simulink model "Copy_of_tests"  (R2024b)
settings: Solver=VariableStepAuto  StartTime=0.0  StopTime=1  RelTol=1e-3  AbsTol=1e-3  EnableMultiTasking=on
values from neighbouring files (symbols this model uses):
  m = obj.Br *obj.volume / obj.mu    [External_Magnet2.m]
  Params = Sim_Param_Setup    [Sim_Open.m]
undefined symbols (not defined in the file or in its folder): X, Y, Z
libraries: sm_lib x171, vrlib x144, nesl_utility x101, matrix_library x91, sharedtransform x12
(part 5 of 9)

== system Copy_of_tests/Multi-Arm system/Single_Arm 1/Plate_2/Torques and Forces ==
  m_slave : Inport
  Pos_Slave : Inport  Port=2
  M1 : Inport  Port=3
  Pos_Plate1 : Inport  Port=4
  M3 : Inport  Port=5
  Pos_Plate3 : Inport  Port=6
  M4 : Inport  Port=7
  Pos_Plate4 : Inport  Port=8
  M5 : Inport  Port=9
  Pos_Plate5 : Inport  Port=10
  M6 : Inport  Port=11
  Pos_Plate6 : Inport  Port=12
  Add{,1..4} (5 alike) : Sum  Inputs=+-
  Magnetic Forces : Subsystem
  Magnetic Torques : Subsystem
      settings: PortSchema="{\"entries\":[{\"content\":{\"sides\":[{\"content\":{\"connectorIds\":[\"In1\",\"In2\",\"In3\",\"In4\",\"In5\",\"In6\",\"In7\",\"In8\",\"In9\",\"In10\",\"In11\"]},\"type\":\"ConnectorPlacement.EquallySpacedRectSide\",\"uuid\":\"6f05c61b-28f4-4565-bbea-1be0fb93c6f0\"},{\"content\":{\"connectorIds\":[\"Out1\"],\"side\":\"RIGHT\"},\"type\":\"ConnectorPlacement.EquallySpacedRectSide\",\"uuid\":\"8634642c-fc93-4182-aaec-4f6aca47cd70\"},{\"content\":{\"connectorIds\":[\"LConn1\"],\"side\":\"TOP\"},\"type\":\"ConnectorPlacement.EquallySpacedRectSide\",\"uuid\":\"4c29c46f-a8de-4915-ac6e-9828579e7b84\"}]},\"type\":\"ConnectorPlacement.EquallySpacedConnector\",\"uuid\":\"3da81916-5d74-4352-a0fa-851a5433a86b\"}],\"packageUris\":[\"http://schema.mathworks.com/mf0/Connector/R2020b\"],\"version\":\"1.0\"}"
  brick reference : PMIOPort  Side=Left
  Forces : Outport
  Torques : Outport  Port=2
  wires:
  m_slave/1 -> Magnetic Forces/1(m_slave), Magnetic Torques/1(m_slave)
  Pos_Slave/1 -> Add4/1, Add3/1, Add2/1, Add1/1, Add/1
  Pos_Plate1/1 -> Add/2
  M1/1 -> Magnetic Torques/2(M1), Magnetic Forces/2(M1)
  Add/1 -> Magnetic Torques/7(r1), Magnetic Forces/7(r1)
  Pos_Plate6/1 -> Add4/2
  Pos_Plate5/1 -> Add3/2
  Pos_Plate4/1 -> Add2/2
  Pos_Plate3/1 -> Add1/2
  M3/1 -> Magnetic Forces/3(M3), Magnetic Torques/3(M3)
  Add1/1 -> Magnetic Torques/8(r3), Magnetic Forces/8(r3)
  M4/1 -> Magnetic Forces/4(M4), Magnetic Torques/4(M4)
  M5/1 -> Magnetic Forces/5(M5), Magnetic Torques/5(M5)
  M6/1 -> Magnetic Forces/6(M6), Magnetic Torques/6(M6)
  Add2/1 -> Magnetic Forces/9(r4), Magnetic Torques/9(r4)
  Add3/1 -> Magnetic Forces/10(r5), Magnetic Torques/10(r5)
  Add4/1 -> Magnetic Forces/11(r6), Magnetic Torques/11(r6)
  Magnetic Forces/1(Forces) -> Forces/1
  Magnetic Torques/1(Torque) -> Torques/1
  connections:
  brick reference/RConn1 -- Magnetic Torques/LConn1

== system Copy_of_tests/Multi-Arm system/Single_Arm 1/Plate_3/Subsystem ==
  Slave_Moment : Inport
  Slave_Pos : Inport  Port=2
  Source_Moment : Inport  Port=3
  Source_Pos : Inport  Port=4
  Add : Sum  Inputs=+-
  Add1 : Sum  Inputs=+-
  Add2 : Sum  Inputs=+-
  Add3 : Sum  Inputs=+++
  Constant : Constant  Value=-3
  Constant1 : Constant  Value=-4
  Cross Product : matrix_library/Cross Product
  Dot Product : DotProduct  OutDataTypeStr=Inherit: Inherit via internal rule
  Dot Product1 : DotProduct  OutDataTypeStr=Inherit: Inherit via internal rule
  Gain : Gain  Gain=4*pi*1e-7/(4*pi)
  Gain1 : Gain  Gain=3
  Gain2 : Gain  Gain=3*4*pi*1e-7/(4*pi)
  Gain3 : Gain  Gain=5
  IdentityMatrix : IdentityMatrix  OutputDimensions=3
  Matrix Multiply : Product  Multiplication=Matrix(*)
  Matrix Multiply1 : Product  Multiplication=Matrix(*)
  Normalize Vector : vrlib/Utilities/Normalize Vector  maxzero=0
  Normalize Vector1 : vrlib/Utilities/Normalize Vector  maxzero=0
  Power : Math  Operator=pow
  Power1 : Math  Operator=pow
  Product{,1..5} (6 alike) : Product
  Sqrt : Sqrt
  Sqrt1 : Sqrt
  Transpose : Math  Operator=transpose
  m dot m : DotProduct  OutDataTypeStr=Inherit: Inherit via internal rule
  r dot m_master : DotProduct  OutDataTypeStr=Inherit: Inherit via internal rule
  r dot m_slave : DotProduct  OutDataTypeStr=Inherit: Inherit via internal rule
  Source_Torque : Outport
  Source_Force : Outport  Port=2
  wires:
  Power/1 -> Gain/1
  Transpose/1 -> Matrix Multiply/2
  Gain1/1 -> Add/1
  Matrix Multiply/1 -> Gain1/1
  Sqrt/1 -> Power/1
  Gain/1 -> Product/2
  Dot Product/1 -> Sqrt/1
  Product/1 -> Cross Product/2
  Matrix Multiply1/1 -> Product/1
  Normalize Vector/1 -> Transpose/1, Matrix Multiply/1
  IdentityMatrix/1 -> Add/2
  Constant/1 -> Power/2
  Add/1 -> Matrix Multiply1/1
  Slave_Pos/1 -> Add1/1
  Source_Pos/1 -> Add1/2
  Cross Product/1 -> Source_Torque/1
  Slave_Moment/1 -> Cross Product/1, Product2/2, m dot m/1, r dot m_slave/2
  Normalize Vector1/1 -> r dot m_slave/1, r dot m_master/1, Product4/2
  Add3/1 -> Product5/2
  Gain2/1 -> Product5/1
  Product4/1 -> Add3/3
  Dot Product1/1 -> Sqrt1/1
  Gain3/1 -> Add2/2
  r dot m_master/1 -> Product3/2, Product2/1
  Source_Moment/1 -> Matrix Multiply1/2, m dot m/2, Product1/2, r dot m_master/2
  m dot m/1 -> Add2/1
  Power1/1 -> Gain2/1
  Sqrt1/1 -> Power1/1
  r dot m_slave/1 -> Product1/1, Product3/1
  Product2/1 -> Add3/2
  Constant1/1 -> Power1/2
  Add2/1 -> Product4/1
  Add1/1 -> Normalize Vector1/1, Dot Product1/2, Dot Product1/1, Dot Product/2, Dot Product/1, Normalize Vector/1
  Product3/1 -> Gain3/1
  Product1/1 -> Add3/1
  Product5/1 -> Source_Force/1

== system Copy_of_tests/Multi-Arm system/Single_Arm 1/Plate_3/Torques and Forces ==
  m_slave : Inport
  Pos_Slave : Inport  Port=2
  M1 : Inport  Port=3
  Pos_Plate1 : Inport  Port=4
  M2 : Inport  Port=5
  Pos_Plate2 : Inport  Port=6
  M4 : Inport  Port=7
  Pos_Plate4 : Inport  Port=8
  M5 : Inport  Port=9
  Pos_Plate5 : Inport  Port=10
  M6 : Inport  Port=11
  Pos_Plate6 : Inport  Port=12
  Add{,1..4} (5 alike) : Sum  Inputs=+-
  Magnetic Forces : Subsystem
  Magnetic Torques : Subsystem
      settings: PortSchema="{\"entries\":[{\"content\":{\"sides\":[{\"content\":{\"connectorIds\":[\"In1\",\"In2\",\"In3\",\"In4\",\"In5\",\"In6\",\"In7\",\"In8\",\"In9\",\"In10\",\"In11\"]},\"type\":\"ConnectorPlacement.EquallySpacedRectSide\",\"uuid\":\"05771496-45a2-4580-b6ab-cadf9064ee26\"},{\"content\":{\"connectorIds\":[\"Out1\"],\"side\":\"RIGHT\"},\"type\":\"ConnectorPlacement.EquallySpacedRectSide\",\"uuid\":\"b79900f2-9f02-4790-af3a-0fbba66daa11\"},{\"content\":{\"connectorIds\":[\"LConn1\"],\"side\":\"TOP\"},\"type\":\"ConnectorPlacement.EquallySpacedRectSide\",\"uuid\":\"95266051-22b3-46d7-add2-de0ce2a92008\"}]},\"type\":\"ConnectorPlacement.EquallySpacedConnector\",\"uuid\":\"2bf1b23d-6512-437d-b945-3c726b6a255c\"}],\"packageUris\":[\"http://schema.mathworks.com/mf0/Connector/R2020b\"],\"version\":\"1.0\"}"
  brick reference : PMIOPort  Side=Left
  Forces : Outport
  Torques : Outport  Port=2
  wires:
  m_slave/1 -> Magnetic Forces/1(m_slave), Magnetic Torques/1(m_slave)
  Pos_Slave/1 -> Add4/1, Add3/1, Add2/1, Add1/1, Add/1
  Pos_Plate1/1 -> Add/2
  M1/1 -> Magnetic Torques/2(M1), Magnetic Forces/2(M1)
  Add/1 -> Magnetic Torques/7(r1), Magnetic Forces/7(r1)
  Pos_Plate6/1 -> Add4/2
  Pos_Plate5/1 -> Add3/2
  Pos_Plate4/1 -> Add2/2
  Pos_Plate2/1 -> Add1/2
  M2/1 -> Magnetic Forces/3(M2), Magnetic Torques/3(M2)
  Add1/1 -> Magnetic Torques/8(r2), Magnetic Forces/8(r2)
  M4/1 -> Magnetic Forces/4(M4), Magnetic Torques/4(M4)
  M5/1 -> Magnetic Forces/5(M5), Magnetic Torques/5(M5)
  M6/1 -> Magnetic Forces/6(M6), Magnetic Torques/6(M6)
  Add2/1 -> Magnetic Forces/9(r4), Magnetic Torques/9(r4)
  Add3/1 -> Magnetic Forces/10(r5), Magnetic Torques/10(r5)
  Add4/1 -> Magnetic Forces/11(r6), Magnetic Torques/11(r6)
  Magnetic Forces/1(Forces) -> Forces/1
  Magnetic Torques/1(Torque) -> Torques/1
  connections:
  brick reference/RConn1 -- Magnetic Torques/LConn1

== system Copy_of_tests/Multi-Arm system/Single_Arm 1/Plate_4/Subsystem ==
  Slave_Moment : Inport
  Slave_Pos : Inport  Port=2
  Source_Moment : Inport  Port=3
  Source_Pos : Inport  Port=4
  Add : Sum  Inputs=+-
  Add1 : Sum  Inputs=+-
  Add2 : Sum  Inputs=+-
  Add3 : Sum  Inputs=+++
  Constant : Constant  Value=-3
  Constant1 : Constant  Value=-4
  Cross Product : matrix_library/Cross Product
  Dot Product : DotProduct  OutDataTypeStr=Inherit: Inherit via internal rule
  Dot Product1 : DotProduct  OutDataTypeStr=Inherit: Inherit via internal rule
  Gain : Gain  Gain=4*pi*1e-7/(4*pi)
  Gain1 : Gain  Gain=3
  Gain2 : Gain  Gain=3*4*pi*1e-7/(4*pi)
  Gain3 : Gain  Gain=5
  IdentityMatrix : IdentityMatrix  OutputDimensions=3
  Matrix Multiply : Product  Multiplication=Matrix(*)
  Matrix Multiply1 : Product  Multiplication=Matrix(*)
  Normalize Vector : vrlib/Utilities/Normalize Vector  maxzero=0
  Normalize Vector1 : vrlib/Utilities/Normalize Vector  maxzero=0
  Power : Math  Operator=pow
  Power1 : Math  Operator=pow
  Product{,1..5} (6 alike) : Product
  Sqrt : Sqrt
  Sqrt1 : Sqrt
  Transpose : Math  Operator=transpose
  m dot m : DotProduct  OutDataTypeStr=Inherit: Inherit via internal rule
  r dot m_master : DotProduct  OutDataTypeStr=Inherit: Inherit via internal rule
  r dot m_slave : DotProduct  OutDataTypeStr=Inherit: Inherit via internal rule
  Source_Torque : Outport
  Source_Force : Outport  Port=2
  wires:
  Power/1 -> Gain/1
  Transpose/1 -> Matrix Multiply/2
  Gain1/1 -> Add/1
  Matrix Multiply/1 -> Gain1/1
  Sqrt/1 -> Power/1
  Gain/1 -> Product/2
  Dot Product/1 -> Sqrt/1
  Product/1 -> Cross Product/2
  Matrix Multiply1/1 -> Product/1
  Normalize Vector/1 -> Transpose/1, Matrix Multiply/1
  IdentityMatrix/1 -> Add/2
  Constant/1 -> Power/2
  Add/1 -> Matrix Multiply1/1
  Slave_Pos/1 -> Add1/1
  Source_Pos/1 -> Add1/2
  Cross Product/1 -> Source_Torque/1
  Slave_Moment/1 -> Cross Product/1, Product2/2, m dot m/1, r dot m_slave/2
  Normalize Vector1/1 -> r dot m_slave/1, r dot m_master/1, Product4/2
  Add3/1 -> Product5/2
  Gain2/1 -> Product5/1
  Product4/1 -> Add3/3
  Dot Product1/1 -> Sqrt1/1
  Gain3/1 -> Add2/2
  r dot m_master/1 -> Product3/2, Product2/1
  Source_Moment/1 -> Matrix Multiply1/2, m dot m/2, Product1/2, r dot m_master/2
  m dot m/1 -> Add2/1
  Power1/1 -> Gain2/1
  Sqrt1/1 -> Power1/1
  r dot m_slave/1 -> Product1/1, Product3/1
  Product2/1 -> Add3/2
  Constant1/1 -> Power1/2
  Add2/1 -> Product4/1
  Add1/1 -> Normalize Vector1/1, Dot Product1/2, Dot Product1/1, Dot Product/2, Dot Product/1, Normalize Vector/1
  Product3/1 -> Gain3/1
  Product1/1 -> Add3/1
  Product5/1 -> Source_Force/1

== system Copy_of_tests/Multi-Arm system/Single_Arm 1/Plate_4/Torques and Forces ==
  m_slave : Inport
  Pos_Slave : Inport  Port=2
  M1 : Inport  Port=3
  Pos_Plate1 : Inport  Port=4
  M2 : Inport  Port=5
  Pos_Plate2 : Inport  Port=6
  M3 : Inport  Port=7
  Pos_Plate3 : Inport  Port=8
  M5 : Inport  Port=9
  Pos_Plate5 : Inport  Port=10
  M6 : Inport  Port=11
  Pos_Plate6 : Inport  Port=12
  Add{,1..4} (5 alike) : Sum  Inputs=+-
  Magnetic Forces : Subsystem
  Magnetic Torques : Subsystem
      settings: PortSchema="{\"entries\":[{\"content\":{\"sides\":[{\"content\":{\"connectorIds\":[\"In1\",\"In2\",\"In3\",\"In4\",\"In5\",\"In6\",\"In7\",\"In8\",\"In9\",\"In10\",\"In11\"]},\"type\":\"ConnectorPlacement.EquallySpacedRectSide\",\"uuid\":\"05771496-45a2-4580-b6ab-cadf9064ee26\"},{\"content\":{\"connectorIds\":[\"Out1\"],\"side\":\"RIGHT\"},\"type\":\"ConnectorPlacement.EquallySpacedRectSide\",\"uuid\":\"b79900f2-9f02-4790-af3a-0fbba66daa11\"},{\"content\":{\"connectorIds\":[\"LConn1\"],\"side\":\"TOP\"},\"type\":\"ConnectorPlacement.EquallySpacedRectSide\",\"uuid\":\"95266051-22b3-46d7-add2-de0ce2a92008\"}]},\"type\":\"ConnectorPlacement.EquallySpacedConnector\",\"uuid\":\"2bf1b23d-6512-437d-b945-3c726b6a255c\"}],\"packageUris\":[\"http://schema.mathworks.com/mf0/Connector/R2020b\"],\"version\":\"1.0\"}"
  brick reference : PMIOPort  Side=Left
  Forces : Outport
  Torques : Outport  Port=2
  wires:
  m_slave/1 -> Magnetic Forces/1(m_slave), Magnetic Torques/1(m_slave)
  Pos_Slave/1 -> Add4/1, Add3/1, Add2/1, Add1/1, Add/1
  Pos_Plate1/1 -> Add/2
  M1/1 -> Magnetic Torques/2(M1), Magnetic Forces/2(M1)
  Add/1 -> Magnetic Torques/7(r1), Magnetic Forces/7(r1)
  Pos_Plate6/1 -> Add4/2
  Pos_Plate5/1 -> Add3/2
  Pos_Plate3/1 -> Add2/2
  Pos_Plate2/1 -> Add1/2
  M2/1 -> Magnetic Forces/3(M2), Magnetic Torques/3(M2)
  Add1/1 -> Magnetic Torques/8(r2), Magnetic Forces/8(r2)
  M3/1 -> Magnetic Forces/4(M3), Magnetic Torques/4(M3)
  M5/1 -> Magnetic Forces/5(M5), Magnetic Torques/5(M5)
  M6/1 -> Magnetic Forces/6(M6), Magnetic Torques/6(M6)
  Add2/1 -> Magnetic Forces/9(r3), Magnetic Torques/9(r3)
  Add3/1 -> Magnetic Forces/10(r5), Magnetic Torques/10(r5)
  Add4/1 -> Magnetic Forces/11(r6), Magnetic Torques/11(r6)
  Magnetic Forces/1(Forces) -> Forces/1
  Magnetic Torques/1(Torque) -> Torques/1
  connections:
  brick reference/RConn1 -- Magnetic Torques/LConn1

== system Copy_of_tests/Multi-Arm system/Single_Arm 1/Plate_5/Subsystem ==
  Slave_Moment : Inport
  Slave_Pos : Inport  Port=2
  Source_Moment : Inport  Port=3
  Source_Pos : Inport  Port=4
  Add : Sum  Inputs=+-
  Add1 : Sum  Inputs=+-
  Add2 : Sum  Inputs=+-
  Add3 : Sum  Inputs=+++
  Constant : Constant  Value=-3
  Constant1 : Constant  Value=-4
  Cross Product : matrix_library/Cross Product
  Dot Product : DotProduct  OutDataTypeStr=Inherit: Inherit via internal rule
  Dot Product1 : DotProduct  OutDataTypeStr=Inherit: Inherit via internal rule
  Gain : Gain  Gain=4*pi*1e-7/(4*pi)
  Gain1 : Gain  Gain=3
  Gain2 : Gain  Gain=3*4*pi*1e-7/(4*pi)
  Gain3 : Gain  Gain=5
  IdentityMatrix : IdentityMatrix  OutputDimensions=3
  Matrix Multiply : Product  Multiplication=Matrix(*)
  Matrix Multiply1 : Product  Multiplication=Matrix(*)
  Normalize Vector : vrlib/Utilities/Normalize Vector  maxzero=0
  Normalize Vector1 : vrlib/Utilities/Normalize Vector  maxzero=0
  Power : Math  Operator=pow
  Power1 : Math  Operator=pow
  Product{,1..5} (6 alike) : Product
  Sqrt : Sqrt
  Sqrt1 : Sqrt
  Transpose : Math  Operator=transpose
  m dot m : DotProduct  OutDataTypeStr=Inherit: Inherit via internal rule
  r dot m_master : DotProduct  OutDataTypeStr=Inherit: Inherit via internal rule
  r dot m_slave : DotProduct  OutDataTypeStr=Inherit: Inherit via internal rule
  Source_Torque : Outport
  Source_Force : Outport  Port=2
  wires:
  Power/1 -> Gain/1
  Transpose/1 -> Matrix Multiply/2
  Gain1/1 -> Add/1
  Matrix Multiply/1 -> Gain1/1
  Sqrt/1 -> Power/1
  Gain/1 -> Product/2
  Dot Product/1 -> Sqrt/1
  Product/1 -> Cross Product/2
  Matrix Multiply1/1 -> Product/1
  Normalize Vector/1 -> Transpose/1, Matrix Multiply/1
  IdentityMatrix/1 -> Add/2
  Constant/1 -> Power/2
  Add/1 -> Matrix Multiply1/1
  Slave_Pos/1 -> Add1/1
  Source_Pos/1 -> Add1/2
  Cross Product/1 -> Source_Torque/1
  Slave_Moment/1 -> Cross Product/1, Product2/2, m dot m/1, r dot m_slave/2
  Normalize Vector1/1 -> r dot m_slave/1, r dot m_master/1, Product4/2
  Add3/1 -> Product5/2
  Gain2/1 -> Product5/1
  Product4/1 -> Add3/3
  Dot Product1/1 -> Sqrt1/1
  Gain3/1 -> Add2/2
  r dot m_master/1 -> Product3/2, Product2/1
  Source_Moment/1 -> Matrix Multiply1/2, m dot m/2, Product1/2, r dot m_master/2
  m dot m/1 -> Add2/1
  Power1/1 -> Gain2/1
  Sqrt1/1 -> Power1/1
  r dot m_slave/1 -> Product1/1, Product3/1
  Product2/1 -> Add3/2
  Constant1/1 -> Power1/2
  Add2/1 -> Product4/1
  Add1/1 -> Normalize Vector1/1, Dot Product1/2, Dot Product1/1, Dot Product/2, Dot Product/1, Normalize Vector/1
  Product3/1 -> Gain3/1
  Product1/1 -> Add3/1
  Product5/1 -> Source_Force/1

== system Copy_of_tests/Multi-Arm system/Single_Arm 1/Plate_5/Torques and Forces ==
  m_slave : Inport
  Pos_Slave : Inport  Port=2
  M1 : Inport  Port=3
  Pos_Plate1 : Inport  Port=4
  M2 : Inport  Port=5
  Pos_Plate2 : Inport  Port=6
  M3 : Inport  Port=7
  Pos_Plate3 : Inport  Port=8
  M4 : Inport  Port=9
  Pos_Plate4 : Inport  Port=10
  M6 : Inport  Port=11
  Pos_Plate6 : Inport  Port=12
  Add{,1..4} (5 alike) : Sum  Inputs=+-
  Magnetic Forces : Subsystem
  Magnetic Torques : Subsystem
      settings: PortSchema="{\"entries\":[{\"content\":{\"sides\":[{\"content\":{\"connectorIds\":[\"In1\",\"In2\",\"In3\",\"In4\",\"In5\",\"In6\",\"In7\",\"In8\",\"In9\",\"In10\",\"In11\"]},\"type\":\"ConnectorPlacement.EquallySpacedRectSide\",\"uuid\":\"05771496-45a2-4580-b6ab-cadf9064ee26\"},{\"content\":{\"connectorIds\":[\"Out1\"],\"side\":\"RIGHT\"},\"type\":\"ConnectorPlacement.EquallySpacedRectSide\",\"uuid\":\"b79900f2-9f02-4790-af3a-0fbba66daa11\"},{\"content\":{\"connectorIds\":[\"LConn1\"],\"side\":\"TOP\"},\"type\":\"ConnectorPlacement.EquallySpacedRectSide\",\"uuid\":\"95266051-22b3-46d7-add2-de0ce2a92008\"}]},\"type\":\"ConnectorPlacement.EquallySpacedConnector\",\"uuid\":\"2bf1b23d-6512-437d-b945-3c726b6a255c\"}],\"packageUris\":[\"http://schema.mathworks.com/mf0/Connector/R2020b\"],\"version\":\"1.0\"}"
  brick reference : PMIOPort  Side=Left
  Forces : Outport
  Torques : Outport  Port=2
  wires:
  m_slave/1 -> Magnetic Forces/1(m_slave), Magnetic Torques/1(m_slave)
  Pos_Slave/1 -> Add4/1, Add3/1, Add2/1, Add1/1, Add/1
  Pos_Plate1/1 -> Add/2
  M1/1 -> Magnetic Torques/2(M1), Magnetic Forces/2(M1)
  Add/1 -> Magnetic Torques/7(r1), Magnetic Forces/7(r1)
  Pos_Plate6/1 -> Add4/2
  Pos_Plate4/1 -> Add3/2
  Pos_Plate3/1 -> Add2/2
  Pos_Plate2/1 -> Add1/2
  M2/1 -> Magnetic Forces/3(M2), Magnetic Torques/3(M2)
  Add1/1 -> Magnetic Torques/8(r2), Magnetic Forces/8(r2)
  M3/1 -> Magnetic Forces/4(M3), Magnetic Torques/4(M3)
  M4/1 -> Magnetic Forces/5(M4), Magnetic Torques/5(M4)
  M6/1 -> Magnetic Forces/6(M6), Magnetic Torques/6(M6)
  Add2/1 -> Magnetic Forces/9(r3), Magnetic Torques/9(r3)
  Add3/1 -> Magnetic Forces/10(r4), Magnetic Torques/10(r4)
  Add4/1 -> Magnetic Forces/11(r6), Magnetic Torques/11(r6)
  Magnetic Forces/1(Forces) -> Forces/1
  Magnetic Torques/1(Torque) -> Torques/1
  connections:
  brick reference/RConn1 -- Magnetic Torques/LConn1

== system Copy_of_tests/Multi-Arm system/Single_Arm 1/Plate_6/Subsystem ==
  Slave_Moment : Inport
  Slave_Pos : Inport  Port=2
  Source_Moment : Inport  Port=3
  Source_Pos : Inport  Port=4
  Add : Sum  Inputs=+-
  Add1 : Sum  Inputs=+-
  Add2 : Sum  Inputs=+-
  Add3 : Sum  Inputs=+++
  Constant : Constant  Value=-3
  Constant1 : Constant  Value=-4
  Cross Product : matrix_library/Cross Product
  Dot Product : DotProduct  OutDataTypeStr=Inherit: Inherit via internal rule
  Dot Product1 : DotProduct  OutDataTypeStr=Inherit: Inherit via internal rule
  Gain : Gain  Gain=4*pi*1e-7/(4*pi)
  Gain1 : Gain  Gain=3
  Gain2 : Gain  Gain=3*4*pi*1e-7/(4*pi)
  Gain3 : Gain  Gain=5
  IdentityMatrix : IdentityMatrix  OutputDimensions=3
  Matrix Multiply : Product  Multiplication=Matrix(*)
  Matrix Multiply1 : Product  Multiplication=Matrix(*)
  Normalize Vector : vrlib/Utilities/Normalize Vector  maxzero=0
  Normalize Vector1 : vrlib/Utilities/Normalize Vector  maxzero=0
  Power : Math  Operator=pow
  Power1 : Math  Operator=pow
  Product{,1..5} (6 alike) : Product
  Sqrt : Sqrt
  Sqrt1 : Sqrt
  Transpose : Math  Operator=transpose
  m dot m : DotProduct  OutDataTypeStr=Inherit: Inherit via internal rule
  r dot m_master : DotProduct  OutDataTypeStr=Inherit: Inherit via internal rule
  r dot m_slave : DotProduct  OutDataTypeStr=Inherit: Inherit via internal rule
  Source_Torque : Outport
  Source_Force : Outport  Port=2
  wires:
  Power/1 -> Gain/1
  Transpose/1 -> Matrix Multiply/2
  Gain1/1 -> Add/1
  Matrix Multiply/1 -> Gain1/1
  Sqrt/1 -> Power/1
  Gain/1 -> Product/2
  Dot Product/1 -> Sqrt/1
  Product/1 -> Cross Product/2
  Matrix Multiply1/1 -> Product/1
  Normalize Vector/1 -> Transpose/1, Matrix Multiply/1
  IdentityMatrix/1 -> Add/2
  Constant/1 -> Power/2
  Add/1 -> Matrix Multiply1/1
  Slave_Pos/1 -> Add1/1
  Source_Pos/1 -> Add1/2
  Cross Product/1 -> Source_Torque/1
  Slave_Moment/1 -> Cross Product/1, Product2/2, m dot m/1, r dot m_slave/2
  Normalize Vector1/1 -> r dot m_slave/1, r dot m_master/1, Product4/2
  Add3/1 -> Product5/2
  Gain2/1 -> Product5/1
  Product4/1 -> Add3/3
  Dot Product1/1 -> Sqrt1/1
  Gain3/1 -> Add2/2
  r dot m_master/1 -> Product3/2, Product2/1
  Source_Moment/1 -> Matrix Multiply1/2, m dot m/2, Product1/2, r dot m_master/2
  m dot m/1 -> Add2/1
  Power1/1 -> Gain2/1
  Sqrt1/1 -> Power1/1
  r dot m_slave/1 -> Product1/1, Product3/1
  Product2/1 -> Add3/2
  Constant1/1 -> Power1/2
  Add2/1 -> Product4/1
  Add1/1 -> Normalize Vector1/1, Dot Product1/2, Dot Product1/1, Dot Product/2, Dot Product/1, Normalize Vector/1
  Product3/1 -> Gain3/1
  Product1/1 -> Add3/1
  Product5/1 -> Source_Force/1

== system Copy_of_tests/Multi-Arm system/Single_Arm 1/Plate_6/Torques and Forces ==
  m_slave : Inport
  Pos_Slave : Inport  Port=2
  M1 : Inport  Port=3
  Pos_Plate1 : Inport  Port=4
  M2 : Inport  Port=5
  Pos_Plate2 : Inport  Port=6
  M3 : Inport  Port=7
  Pos_Plate3 : Inport  Port=8
  M4 : Inport  Port=9
  Pos_Plate4 : Inport  Port=10
  M5 : Inport  Port=11
  Pos_Plate5 : Inport  Port=12
  Add{,1..4} (5 alike) : Sum  Inputs=+-
  Magnetic Forces : Subsystem
  Magnetic Torques : Subsystem
      settings: PortSchema="{\"entries\":[{\"content\":{\"sides\":[{\"content\":{\"connectorIds\":[\"In1\",\"In2\",\"In3\",\"In4\",\"In5\",\"In6\",\"In7\",\"In8\",\"In9\",\"In10\",\"In11\"]},\"type\":\"ConnectorPlacement.EquallySpacedRectSide\",\"uuid\":\"6f05c61b-28f4-4565-bbea-1be0fb93c6f0\"},{\"content\":{\"connectorIds\":[\"Out1\"],\"side\":\"RIGHT\"},\"type\":\"ConnectorPlacement.EquallySpacedRectSide\",\"uuid\":\"8634642c-fc93-4182-aaec-4f6aca47cd70\"},{\"content\":{\"connectorIds\":[\"LConn1\"],\"side\":\"TOP\"},\"type\":\"ConnectorPlacement.EquallySpacedRectSide\",\"uuid\":\"4c29c46f-a8de-4915-ac6e-9828579e7b84\"}]},\"type\":\"ConnectorPlacement.EquallySpacedConnector\",\"uuid\":\"3da81916-5d74-4352-a0fa-851a5433a86b\"}],\"packageUris\":[\"http://schema.mathworks.com/mf0/Connector/R2020b\"],\"version\":\"1.0\"}"
  Brick reference : PMIOPort  Side=Left
  Forces : Outport
  Torques : Outport  Port=2
  wires:
  m_slave/1 -> Magnetic Forces/1(m_slave), Magnetic Torques/1(m_slave)
  Pos_Slave/1 -> Add4/1, Add3/1, Add2/1, Add1/1, Add/1
  Pos_Plate1/1 -> Add/2
  M1/1 -> Magnetic Torques/2(M1), Magnetic Forces/2(M1)
  Add/1 -> Magnetic Torques/7(r1), Magnetic Forces/7(r1)
  Pos_Plate5/1 -> Add4/2
  Pos_Plate4/1 -> Add3/2
  Pos_Plate3/1 -> Add2/2
  Pos_Plate2/1 -> Add1/2
  M2/1 -> Magnetic Forces/3(M2), Magnetic Torques/3(M2)
  Add1/1 -> Magnetic Torques/8(r2), Magnetic Forces/8(r2)
  M3/1 -> Magnetic Forces/4(M3), Magnetic Torques/4(M3)
  M4/1 -> Magnetic Forces/5(M4), Magnetic Torques/5(M4)
  M5/1 -> Magnetic Forces/6(M5), Magnetic Torques/6(M5)
  Add2/1 -> Magnetic Forces/9(r3), Magnetic Torques/9(r3)
  Add3/1 -> Magnetic Forces/10(r4), Magnetic Torques/10(r4)
  Add4/1 -> Magnetic Forces/11(r5), Magnetic Torques/11(r5)
  Magnetic Forces/1(Forces) -> Forces/1
  Magnetic Torques/1(Torque) -> Torques/1
  connections:
  Brick reference/RConn1 -- Magnetic Torques/LConn1

== system Copy_of_tests/Multi-Arm system/Single_Arm 2/Plate_1/Subsystem ==
  Slave_Moment : Inport
  Slave_Pos : Inport  Port=2
  Source_Moment : Inport  Port=3
  Source_Pos : Inport  Port=4
  Add : Sum  Inputs=+-
  Add1 : Sum  Inputs=+-
  Add2 : Sum  Inputs=+-
  Add3 : Sum  Inputs=+++
  Constant : Constant  Value=-3
  Constant1 : Constant  Value=-4
  Cross Product : matrix_library/Cross Product
  Dot Product : DotProduct  OutDataTypeStr=Inherit: Inherit via internal rule
  Dot Product1 : DotProduct  OutDataTypeStr=Inherit: Inherit via internal rule
  Gain : Gain  Gain=4*pi*1e-7/(4*pi)
  Gain1 : Gain  Gain=3
  Gain2 : Gain  Gain=3*4*pi*1e-7/(4*pi)
  Gain3 : Gain  Gain=5
  IdentityMatrix : IdentityMatrix  OutputDimensions=3
  Matrix Multiply : Product  Multiplication=Matrix(*)
  Matrix Multiply1 : Product  Multiplication=Matrix(*)
  Normalize Vector : vrlib/Utilities/Normalize Vector  maxzero=0
  Normalize Vector1 : vrlib/Utilities/Normalize Vector  maxzero=0
  Power : Math  Operator=pow
  Power1 : Math  Operator=pow
  Product{,1..5} (6 alike) : Product
  Sqrt : Sqrt
  Sqrt1 : Sqrt
  Transpose : Math  Operator=transpose
  m dot m : DotProduct  OutDataTypeStr=Inherit: Inherit via internal rule
  r dot m_master : DotProduct  OutDataTypeStr=Inherit: Inherit via internal rule
  r dot m_slave : DotProduct  OutDataTypeStr=Inherit: Inherit via internal rule
  Source_Torque : Outport
  Source_Force : Outport  Port=2
  wires:
  Power/1 -> Gain/1
  Transpose/1 -> Matrix Multiply/2
  Gain1/1 -> Add/1
  Matrix Multiply/1 -> Gain1/1
  Sqrt/1 -> Power/1
  Gain/1 -> Product/2
  Dot Product/1 -> Sqrt/1
  Product/1 -> Cross Product/2
  Matrix Multiply1/1 -> Product/1
  Normalize Vector/1 -> Transpose/1, Matrix Multiply/1
  IdentityMatrix/1 -> Add/2
  Constant/1 -> Power/2
  Add/1 -> Matrix Multiply1/1
  Slave_Pos/1 -> Add1/1
  Source_Pos/1 -> Add1/2
  Cross Product/1 -> Source_Torque/1
  Slave_Moment/1 -> Cross Product/1, Product2/2, m dot m/1, r dot m_slave/2
  Normalize Vector1/1 -> r dot m_slave/1, r dot m_master/1, Product4/2
  Add3/1 -> Product5/2
  Gain2/1 -> Product5/1
  Product4/1 -> Add3/3
  Dot Product1/1 -> Sqrt1/1
  Gain3/1 -> Add2/2
  r dot m_master/1 -> Product3/2, Product2/1
  Source_Moment/1 -> Matrix Multiply1/2, m dot m/2, Product1/2, r dot m_master/2
  m dot m/1 -> Add2/1
  Power1/1 -> Gain2/1
  Sqrt1/1 -> Power1/1
  r dot m_slave/1 -> Product1/1, Product3/1
  Product2/1 -> Add3/2
  Constant1/1 -> Power1/2
  Add2/1 -> Product4/1
  Add1/1 -> Normalize Vector1/1, Dot Product1/2, Dot Product1/1, Dot Product/2, Dot Product/1, Normalize Vector/1
  Product3/1 -> Gain3/1
  Product1/1 -> Add3/1
  Product5/1 -> Source_Force/1

== system Copy_of_tests/Multi-Arm system/Single_Arm 2/Plate_1/Torques and Forces ==
  m_slave : Inport
  Pos_Slave : Inport  Port=2
  M2 : Inport  Port=3
  Pos_Plate2 : Inport  Port=4
  M3 : Inport  Port=5
  Pos_Plate3 : Inport  Port=6
  M4 : Inport  Port=7
  Pos_Plate4 : Inport  Port=8
  M5 : Inport  Port=9
  Pos_Plate5 : Inport  Port=10
  M6 : Inport  Port=11
  Pos_Plate6 : Inport  Port=12
  Add{,1..4} (5 alike) : Sum  Inputs=+-
  Magnetic Forces : Subsystem
  Magnetic Torques : Subsystem
      settings: PortSchema="{\"entries\":[{\"content\":{\"sides\":[{\"content\":{\"connectorIds\":[\"In1\",\"In2\",\"In3\",\"In4\",\"In5\",\"In6\",\"In7\",\"In8\",\"In9\",\"In10\",\"In11\"]},\"type\":\"ConnectorPlacement.EquallySpacedRectSide\",\"uuid\":\"6f05c61b-28f4-4565-bbea-1be0fb93c6f0\"},{\"content\":{\"connectorIds\":[\"Out1\"],\"side\":\"RIGHT\"},\"type\":\"ConnectorPlacement.EquallySpacedRectSide\",\"uuid\":\"8634642c-fc93-4182-aaec-4f6aca47cd70\"},{\"content\":{\"connectorIds\":[\"LConn1\"],\"side\":\"TOP\"},\"type\":\"ConnectorPlacement.EquallySpacedRectSide\",\"uuid\":\"4c29c46f-a8de-4915-ac6e-9828579e7b84\"}]},\"type\":\"ConnectorPlacement.EquallySpacedConnector\",\"uuid\":\"3da81916-5d74-4352-a0fa-851a5433a86b\"}],\"packageUris\":[\"http://schema.mathworks.com/mf0/Connector/R2020b\"],\"version\":\"1.0\"}"
  brick reference : PMIOPort  Side=Left
  Forces : Outport
  Torques : Outport  Port=2
  wires:
  m_slave/1 -> Magnetic Forces/1(m_slave), Magnetic Torques/1(m_slave)
  Pos_Slave/1 -> Add4/1, Add3/1, Add2/1, Add1/1, Add/1
  Pos_Plate2/1 -> Add/2
  M2/1 -> Magnetic Torques/2(M2), Magnetic Forces/2(M2)
  Add/1 -> Magnetic Torques/7(r2), Magnetic Forces/7(r2)
  Pos_Plate6/1 -> Add4/2
  Pos_Plate5/1 -> Add3/2
  Pos_Plate4/1 -> Add2/2
  Pos_Plate3/1 -> Add1/2
  M3/1 -> Magnetic Forces/3(M3), Magnetic Torques/3(M3)
  Add1/1 -> Magnetic Torques/8(r3), Magnetic Forces/8(r3)
  M4/1 -> Magnetic Forces/4(M4), Magnetic Torques/4(M4)
  M5/1 -> Magnetic Forces/5(M5), Magnetic Torques/5(M5)
  M6/1 -> Magnetic Forces/6(M6), Magnetic Torques/6(M6)
  Add2/1 -> Magnetic Forces/9(r4), Magnetic Torques/9(r4)
  Add3/1 -> Magnetic Forces/10(r5), Magnetic Torques/10(r5)
  Add4/1 -> Magnetic Forces/11(r6), Magnetic Torques/11(r6)
  Magnetic Forces/1(Forces) -> Forces/1
  Magnetic Torques/1(Torque) -> Torques/1
  connections:
  brick reference/RConn1 -- Magnetic Torques/LConn1

== system Copy_of_tests/Multi-Arm system/Single_Arm 2/Plate_2/Subsystem ==
  Slave_Moment : Inport
  Slave_Pos : Inport  Port=2
  Source_Moment : Inport  Port=3
  Source_Pos : Inport  Port=4
  Add : Sum  Inputs=+-
  Add1 : Sum  Inputs=+-
  Add2 : Sum  Inputs=+-
  Add3 : Sum  Inputs=+++
  Constant : Constant  Value=-3
  Constant1 : Constant  Value=-4
  Cross Product : matrix_library/Cross Product
  Dot Product : DotProduct  OutDataTypeStr=Inherit: Inherit via internal rule
  Dot Product1 : DotProduct  OutDataTypeStr=Inherit: Inherit via internal rule
  Gain : Gain  Gain=4*pi*1e-7/(4*pi)
  Gain1 : Gain  Gain=3
  Gain2 : Gain  Gain=3*4*pi*1e-7/(4*pi)
  Gain3 : Gain  Gain=5
  IdentityMatrix : IdentityMatrix  OutputDimensions=3
  Matrix Multiply : Product  Multiplication=Matrix(*)
  Matrix Multiply1 : Product  Multiplication=Matrix(*)
  Normalize Vector : vrlib/Utilities/Normalize Vector  maxzero=0
  Normalize Vector1 : vrlib/Utilities/Normalize Vector  maxzero=0
  Power : Math  Operator=pow
  Power1 : Math  Operator=pow
  Product{,1..5} (6 alike) : Product
  Sqrt : Sqrt
  Sqrt1 : Sqrt
  Transpose : Math  Operator=transpose
  m dot m : DotProduct  OutDataTypeStr=Inherit: Inherit via internal rule
  r dot m_master : DotProduct  OutDataTypeStr=Inherit: Inherit via internal rule
  r dot m_slave : DotProduct  OutDataTypeStr=Inherit: Inherit via internal rule
  Source_Torque : Outport
  Source_Force : Outport  Port=2
  wires:
  Power/1 -> Gain/1
  Transpose/1 -> Matrix Multiply/2
  Gain1/1 -> Add/1
  Matrix Multiply/1 -> Gain1/1
  Sqrt/1 -> Power/1
  Gain/1 -> Product/2
  Dot Product/1 -> Sqrt/1
  Product/1 -> Cross Product/2
  Matrix Multiply1/1 -> Product/1
  Normalize Vector/1 -> Transpose/1, Matrix Multiply/1
  IdentityMatrix/1 -> Add/2
  Constant/1 -> Power/2
  Add/1 -> Matrix Multiply1/1
  Slave_Pos/1 -> Add1/1
  Source_Pos/1 -> Add1/2
  Cross Product/1 -> Source_Torque/1
  Slave_Moment/1 -> Cross Product/1, Product2/2, m dot m/1, r dot m_slave/2
  Normalize Vector1/1 -> r dot m_slave/1, r dot m_master/1, Product4/2
  Add3/1 -> Product5/2
  Gain2/1 -> Product5/1
  Product4/1 -> Add3/3
  Dot Product1/1 -> Sqrt1/1
  Gain3/1 -> Add2/2
  r dot m_master/1 -> Product3/2, Product2/1
  Source_Moment/1 -> Matrix Multiply1/2, m dot m/2, Product1/2, r dot m_master/2
  m dot m/1 -> Add2/1
  Power1/1 -> Gain2/1
  Sqrt1/1 -> Power1/1
  r dot m_slave/1 -> Product1/1, Product3/1
  Product2/1 -> Add3/2
  Constant1/1 -> Power1/2
  Add2/1 -> Product4/1
  Add1/1 -> Normalize Vector1/1, Dot Product1/2, Dot Product1/1, Dot Product/2, Dot Product/1, Normalize Vector/1
  Product3/1 -> Gain3/1
  Product1/1 -> Add3/1
  Product5/1 -> Source_Force/1

== system Copy_of_tests/Multi-Arm system/Single_Arm 2/Plate_2/Torques and Forces ==
  m_slave : Inport
  Pos_Slave : Inport  Port=2
  M1 : Inport  Port=3
  Pos_Plate1 : Inport  Port=4
  M3 : Inport  Port=5
  Pos_Plate3 : Inport  Port=6
  M4 : Inport  Port=7
  Pos_Plate4 : Inport  Port=8
  M5 : Inport  Port=9
  Pos_Plate5 : Inport  Port=10
  M6 : Inport  Port=11
  Pos_Plate6 : Inport  Port=12
  Add{,1..4} (5 alike) : Sum  Inputs=+-
  Magnetic Forces : Subsystem
  Magnetic Torques : Subsystem
      settings: PortSchema="{\"entries\":[{\"content\":{\"sides\":[{\"content\":{\"connectorIds\":[\"In1\",\"In2\",\"In3\",\"In4\",\"In5\",\"In6\",\"In7\",\"In8\",\"In9\",\"In10\",\"In11\"]},\"type\":\"ConnectorPlacement.EquallySpacedRectSide\",\"uuid\":\"6f05c61b-28f4-4565-bbea-1be0fb93c6f0\"},{\"content\":{\"connectorIds\":[\"Out1\"],\"side\":\"RIGHT\"},\"type\":\"ConnectorPlacement.EquallySpacedRectSide\",\"uuid\":\"8634642c-fc93-4182-aaec-4f6aca47cd70\"},{\"content\":{\"connectorIds\":[\"LConn1\"],\"side\":\"TOP\"},\"type\":\"ConnectorPlacement.EquallySpacedRectSide\",\"uuid\":\"4c29c46f-a8de-4915-ac6e-9828579e7b84\"}]},\"type\":\"ConnectorPlacement.EquallySpacedConnector\",\"uuid\":\"3da81916-5d74-4352-a0fa-851a5433a86b\"}],\"packageUris\":[\"http://schema.mathworks.com/mf0/Connector/R2020b\"],\"version\":\"1.0\"}"
  brick reference : PMIOPort  Side=Left
  Forces : Outport
  Torques : Outport  Port=2
  wires:
  m_slave/1 -> Magnetic Forces/1(m_slave), Magnetic Torques/1(m_slave)
  Pos_Slave/1 -> Add4/1, Add3/1, Add2/1, Add1/1, Add/1
  Pos_Plate1/1 -> Add/2
  M1/1 -> Magnetic Torques/2(M1), Magnetic Forces/2(M1)
  Add/1 -> Magnetic Torques/7(r1), Magnetic Forces/7(r1)
  Pos_Plate6/1 -> Add4/2
  Pos_Plate5/1 -> Add3/2
  Pos_Plate4/1 -> Add2/2
  Pos_Plate3/1 -> Add1/2
  M3/1 -> Magnetic Forces/3(M3), Magnetic Torques/3(M3)
  Add1/1 -> Magnetic Torques/8(r3), Magnetic Forces/8(r3)
  M4/1 -> Magnetic Forces/4(M4), Magnetic Torques/4(M4)
  M5/1 -> Magnetic Forces/5(M5), Magnetic Torques/5(M5)
  M6/1 -> Magnetic Forces/6(M6), Magnetic Torques/6(M6)
  Add2/1 -> Magnetic Forces/9(r4), Magnetic Torques/9(r4)
  Add3/1 -> Magnetic Forces/10(r5), Magnetic Torques/10(r5)
  Add4/1 -> Magnetic Forces/11(r6), Magnetic Torques/11(r6)
  Magnetic Forces/1(Forces) -> Forces/1
  Magnetic Torques/1(Torque) -> Torques/1
  connections:
  brick reference/RConn1 -- Magnetic Torques/LConn1

== system Copy_of_tests/Multi-Arm system/Single_Arm 2/Plate_3/Subsystem ==
  Slave_Moment : Inport
  Slave_Pos : Inport  Port=2
  Source_Moment : Inport  Port=3
  Source_Pos : Inport  Port=4
  Add : Sum  Inputs=+-
  Add1 : Sum  Inputs=+-
  Add2 : Sum  Inputs=+-
  Add3 : Sum  Inputs=+++
  Constant : Constant  Value=-3
  Constant1 : Constant  Value=-4
  Cross Product : matrix_library/Cross Product
  Dot Product : DotProduct  OutDataTypeStr=Inherit: Inherit via internal rule
  Dot Product1 : DotProduct  OutDataTypeStr=Inherit: Inherit via internal rule
  Gain : Gain  Gain=4*pi*1e-7/(4*pi)
  Gain1 : Gain  Gain=3
  Gain2 : Gain  Gain=3*4*pi*1e-7/(4*pi)
  Gain3 : Gain  Gain=5
  IdentityMatrix : IdentityMatrix  OutputDimensions=3
  Matrix Multiply : Product  Multiplication=Matrix(*)
  Matrix Multiply1 : Product  Multiplication=Matrix(*)
  Normalize Vector : vrlib/Utilities/Normalize Vector  maxzero=0
  Normalize Vector1 : vrlib/Utilities/Normalize Vector  maxzero=0
  Power : Math  Operator=pow
  Power1 : Math  Operator=pow
  Product{,1..5} (6 alike) : Product
  Sqrt : Sqrt
  Sqrt1 : Sqrt
  Transpose : Math  Operator=transpose
  m dot m : DotProduct  OutDataTypeStr=Inherit: Inherit via internal rule
  r dot m_master : DotProduct  OutDataTypeStr=Inherit: Inherit via internal rule
  r dot m_slave : DotProduct  OutDataTypeStr=Inherit: Inherit via internal rule
  Source_Torque : Outport
  Source_Force : Outport  Port=2
  wires:
  Power/1 -> Gain/1
  Transpose/1 -> Matrix Multiply/2
  Gain1/1 -> Add/1
  Matrix Multiply/1 -> Gain1/1
  Sqrt/1 -> Power/1
  Gain/1 -> Product/2
  Dot Product/1 -> Sqrt/1
  Product/1 -> Cross Product/2
  Matrix Multiply1/1 -> Product/1
  Normalize Vector/1 -> Transpose/1, Matrix Multiply/1
  IdentityMatrix/1 -> Add/2
  Constant/1 -> Power/2
  Add/1 -> Matrix Multiply1/1
  Slave_Pos/1 -> Add1/1
  Source_Pos/1 -> Add1/2
  Cross Product/1 -> Source_Torque/1
  Slave_Moment/1 -> Cross Product/1, Product2/2, m dot m/1, r dot m_slave/2
  Normalize Vector1/1 -> r dot m_slave/1, r dot m_master/1, Product4/2
  Add3/1 -> Product5/2
  Gain2/1 -> Product5/1
  Product4/1 -> Add3/3
  Dot Product1/1 -> Sqrt1/1
  Gain3/1 -> Add2/2
  r dot m_master/1 -> Product3/2, Product2/1
  Source_Moment/1 -> Matrix Multiply1/2, m dot m/2, Product1/2, r dot m_master/2
  m dot m/1 -> Add2/1
  Power1/1 -> Gain2/1
  Sqrt1/1 -> Power1/1
  r dot m_slave/1 -> Product1/1, Product3/1
  Product2/1 -> Add3/2
  Constant1/1 -> Power1/2
  Add2/1 -> Product4/1
  Add1/1 -> Normalize Vector1/1, Dot Product1/2, Dot Product1/1, Dot Product/2, Dot Product/1, Normalize Vector/1
  Product3/1 -> Gain3/1
  Product1/1 -> Add3/1
  Product5/1 -> Source_Force/1

== system Copy_of_tests/Multi-Arm system/Single_Arm 2/Plate_3/Torques and Forces ==
  m_slave : Inport
  Pos_Slave : Inport  Port=2
  M1 : Inport  Port=3
  Pos_Plate1 : Inport  Port=4
  M2 : Inport  Port=5
  Pos_Plate2 : Inport  Port=6
  M4 : Inport  Port=7
  Pos_Plate4 : Inport  Port=8
  M5 : Inport  Port=9
  Pos_Plate5 : Inport  Port=10
  M6 : Inport  Port=11
  Pos_Plate6 : Inport  Port=12
  Add{,1..4} (5 alike) : Sum  Inputs=+-
  Magnetic Forces : Subsystem
  Magnetic Torques : Subsystem
      settings: PortSchema="{\"entries\":[{\"content\":{\"sides\":[{\"content\":{\"connectorIds\":[\"In1\",\"In2\",\"In3\",\"In4\",\"In5\",\"In6\",\"In7\",\"In8\",\"In9\",\"In10\",\"In11\"]},\"type\":\"ConnectorPlacement.EquallySpacedRectSide\",\"uuid\":\"05771496-45a2-4580-b6ab-cadf9064ee26\"},{\"content\":{\"connectorIds\":[\"Out1\"],\"side\":\"RIGHT\"},\"type\":\"ConnectorPlacement.EquallySpacedRectSide\",\"uuid\":\"b79900f2-9f02-4790-af3a-0fbba66daa11\"},{\"content\":{\"connectorIds\":[\"LConn1\"],\"side\":\"TOP\"},\"type\":\"ConnectorPlacement.EquallySpacedRectSide\",\"uuid\":\"95266051-22b3-46d7-add2-de0ce2a92008\"}]},\"type\":\"ConnectorPlacement.EquallySpacedConnector\",\"uuid\":\"2bf1b23d-6512-437d-b945-3c726b6a255c\"}],\"packageUris\":[\"http://schema.mathworks.com/mf0/Connector/R2020b\"],\"version\":\"1.0\"}"
  brick reference : PMIOPort  Side=Left
  Forces : Outport
  Torques : Outport  Port=2
  wires:
  m_slave/1 -> Magnetic Forces/1(m_slave), Magnetic Torques/1(m_slave)
  Pos_Slave/1 -> Add4/1, Add3/1, Add2/1, Add1/1, Add/1
  Pos_Plate1/1 -> Add/2
  M1/1 -> Magnetic Torques/2(M1), Magnetic Forces/2(M1)
  Add/1 -> Magnetic Torques/7(r1), Magnetic Forces/7(r1)
  Pos_Plate6/1 -> Add4/2
  Pos_Plate5/1 -> Add3/2
  Pos_Plate4/1 -> Add2/2
  Pos_Plate2/1 -> Add1/2
  M2/1 -> Magnetic Forces/3(M2), Magnetic Torques/3(M2)
  Add1/1 -> Magnetic Torques/8(r2), Magnetic Forces/8(r2)
  M4/1 -> Magnetic Forces/4(M4), Magnetic Torques/4(M4)
  M5/1 -> Magnetic Forces/5(M5), Magnetic Torques/5(M5)
  M6/1 -> Magnetic Forces/6(M6), Magnetic Torques/6(M6)
  Add2/1 -> Magnetic Forces/9(r4), Magnetic Torques/9(r4)
  Add3/1 -> Magnetic Forces/10(r5), Magnetic Torques/10(r5)
  Add4/1 -> Magnetic Forces/11(r6), Magnetic Torques/11(r6)
  Magnetic Forces/1(Forces) -> Forces/1
  Magnetic Torques/1(Torque) -> Torques/1
  connections:
  brick reference/RConn1 -- Magnetic Torques/LConn1

== system Copy_of_tests/Multi-Arm system/Single_Arm 2/Plate_4/Subsystem ==
  Slave_Moment : Inport
  Slave_Pos : Inport  Port=2
  Source_Moment : Inport  Port=3
  Source_Pos : Inport  Port=4
  Add : Sum  Inputs=+-
  Add1 : Sum  Inputs=+-
  Add2 : Sum  Inputs=+-
  Add3 : Sum  Inputs=+++
  Constant : Constant  Value=-3
  Constant1 : Constant  Value=-4
  Cross Product : matrix_library/Cross Product
  Dot Product : DotProduct  OutDataTypeStr=Inherit: Inherit via internal rule
  Dot Product1 : DotProduct  OutDataTypeStr=Inherit: Inherit via internal rule
  Gain : Gain  Gain=4*pi*1e-7/(4*pi)
  Gain1 : Gain  Gain=3
  Gain2 : Gain  Gain=3*4*pi*1e-7/(4*pi)
  Gain3 : Gain  Gain=5
  IdentityMatrix : IdentityMatrix  OutputDimensions=3
  Matrix Multiply : Product  Multiplication=Matrix(*)
  Matrix Multiply1 : Product  Multiplication=Matrix(*)
  Normalize Vector : vrlib/Utilities/Normalize Vector  maxzero=0
  Normalize Vector1 : vrlib/Utilities/Normalize Vector  maxzero=0
  Power : Math  Operator=pow
  Power1 : Math  Operator=pow
  Product{,1..5} (6 alike) : Product
  Sqrt : Sqrt
  Sqrt1 : Sqrt
  Transpose : Math  Operator=transpose
  m dot m : DotProduct  OutDataTypeStr=Inherit: Inherit via internal rule
  r dot m_master : DotProduct  OutDataTypeStr=Inherit: Inherit via internal rule
  r dot m_slave : DotProduct  OutDataTypeStr=Inherit: Inherit via internal rule
  Source_Torque : Outport
  Source_Force : Outport  Port=2
  wires:
  Power/1 -> Gain/1
  Transpose/1 -> Matrix Multiply/2
  Gain1/1 -> Add/1
  Matrix Multiply/1 -> Gain1/1
  Sqrt/1 -> Power/1
  Gain/1 -> Product/2
  Dot Product/1 -> Sqrt/1
  Product/1 -> Cross Product/2
  Matrix Multiply1/1 -> Product/1
  Normalize Vector/1 -> Transpose/1, Matrix Multiply/1
  IdentityMatrix/1 -> Add/2
  Constant/1 -> Power/2
  Add/1 -> Matrix Multiply1/1
  Slave_Pos/1 -> Add1/1
  Source_Pos/1 -> Add1/2
  Cross Product/1 -> Source_Torque/1
  Slave_Moment/1 -> Cross Product/1, Product2/2, m dot m/1, r dot m_slave/2
  Normalize Vector1/1 -> r dot m_slave/1, r dot m_master/1, Product4/2
  Add3/1 -> Product5/2
  Gain2/1 -> Product5/1
  Product4/1 -> Add3/3
  Dot Product1/1 -> Sqrt1/1
  Gain3/1 -> Add2/2
  r dot m_master/1 -> Product3/2, Product2/1
  Source_Moment/1 -> Matrix Multiply1/2, m dot m/2, Product1/2, r dot m_master/2
  m dot m/1 -> Add2/1
  Power1/1 -> Gain2/1
  Sqrt1/1 -> Power1/1
  r dot m_slave/1 -> Product1/1, Product3/1
  Product2/1 -> Add3/2
  Constant1/1 -> Power1/2
  Add2/1 -> Product4/1
  Add1/1 -> Normalize Vector1/1, Dot Product1/2, Dot Product1/1, Dot Product/2, Dot Product/1, Normalize Vector/1
  Product3/1 -> Gain3/1
  Product1/1 -> Add3/1
  Product5/1 -> Source_Force/1

== system Copy_of_tests/Multi-Arm system/Single_Arm 2/Plate_4/Torques and Forces ==
  m_slave : Inport
  Pos_Slave : Inport  Port=2
  M1 : Inport  Port=3
  Pos_Plate1 : Inport  Port=4
  M2 : Inport  Port=5
  Pos_Plate2 : Inport  Port=6
  M3 : Inport  Port=7
  Pos_Plate3 : Inport  Port=8
  M5 : Inport  Port=9
  Pos_Plate5 : Inport  Port=10
  M6 : Inport  Port=11
  Pos_Plate6 : Inport  Port=12
  Add{,1..4} (5 alike) : Sum  Inputs=+-
  Magnetic Forces : Subsystem
  Magnetic Torques : Subsystem
      settings: PortSchema="{\"entries\":[{\"content\":{\"sides\":[{\"content\":{\"connectorIds\":[\"In1\",\"In2\",\"In3\",\"In4\",\"In5\",\"In6\",\"In7\",\"In8\",\"In9\",\"In10\",\"In11\"]},\"type\":\"ConnectorPlacement.EquallySpacedRectSide\",\"uuid\":\"05771496-45a2-4580-b6ab-cadf9064ee26\"},{\"content\":{\"connectorIds\":[\"Out1\"],\"side\":\"RIGHT\"},\"type\":\"ConnectorPlacement.EquallySpacedRectSide\",\"uuid\":\"b79900f2-9f02-4790-af3a-0fbba66daa11\"},{\"content\":{\"connectorIds\":[\"LConn1\"],\"side\":\"TOP\"},\"type\":\"ConnectorPlacement.EquallySpacedRectSide\",\"uuid\":\"95266051-22b3-46d7-add2-de0ce2a92008\"}]},\"type\":\"ConnectorPlacement.EquallySpacedConnector\",\"uuid\":\"2bf1b23d-6512-437d-b945-3c726b6a255c\"}],\"packageUris\":[\"http://schema.mathworks.com/mf0/Connector/R2020b\"],\"version\":\"1.0\"}"
  brick reference : PMIOPort  Side=Left
  Forces : Outport
  Torques : Outport  Port=2
  wires:
  m_slave/1 -> Magnetic Forces/1(m_slave), Magnetic Torques/1(m_slave)
  Pos_Slave/1 -> Add4/1, Add3/1, Add2/1, Add1/1, Add/1
  Pos_Plate1/1 -> Add/2
  M1/1 -> Magnetic Torques/2(M1), Magnetic Forces/2(M1)
  Add/1 -> Magnetic Torques/7(r1), Magnetic Forces/7(r1)
  Pos_Plate6/1 -> Add4/2
  Pos_Plate5/1 -> Add3/2
  Pos_Plate3/1 -> Add2/2
  Pos_Plate2/1 -> Add1/2
  M2/1 -> Magnetic Forces/3(M2), Magnetic Torques/3(M2)
  Add1/1 -> Magnetic Torques/8(r2), Magnetic Forces/8(r2)
  M3/1 -> Magnetic Forces/4(M3), Magnetic Torques/4(M3)
  M5/1 -> Magnetic Forces/5(M5), Magnetic Torques/5(M5)
  M6/1 -> Magnetic Forces/6(M6), Magnetic Torques/6(M6)
  Add2/1 -> Magnetic Forces/9(r3), Magnetic Torques/9(r3)
  Add3/1 -> Magnetic Forces/10(r5), Magnetic Torques/10(r5)
  Add4/1 -> Magnetic Forces/11(r6), Magnetic Torques/11(r6)
  Magnetic Forces/1(Forces) -> Forces/1
  Magnetic Torques/1(Torque) -> Torques/1
  connections:
  brick reference/RConn1 -- Magnetic Torques/LConn1

== system Copy_of_tests/Multi-Arm system/Single_Arm 2/Plate_5/Subsystem ==
  Slave_Moment : Inport
  Slave_Pos : Inport  Port=2
  Source_Moment : Inport  Port=3
  Source_Pos : Inport  Port=4
  Add : Sum  Inputs=+-
  Add1 : Sum  Inputs=+-
  Add2 : Sum  Inputs=+-
  Add3 : Sum  Inputs=+++
  Constant : Constant  Value=-3
  Constant1 : Constant  Value=-4
  Cross Product : matrix_library/Cross Product
  Dot Product : DotProduct  OutDataTypeStr=Inherit: Inherit via internal rule
  Dot Product1 : DotProduct  OutDataTypeStr=Inherit: Inherit via internal rule
  Gain : Gain  Gain=4*pi*1e-7/(4*pi)
  Gain1 : Gain  Gain=3
  Gain2 : Gain  Gain=3*4*pi*1e-7/(4*pi)
  Gain3 : Gain  Gain=5
  IdentityMatrix : IdentityMatrix  OutputDimensions=3
  Matrix Multiply : Product  Multiplication=Matrix(*)
  Matrix Multiply1 : Product  Multiplication=Matrix(*)
  Normalize Vector : vrlib/Utilities/Normalize Vector  maxzero=0
  Normalize Vector1 : vrlib/Utilities/Normalize Vector  maxzero=0
  Power : Math  Operator=pow
  Power1 : Math  Operator=pow
  Product{,1..5} (6 alike) : Product
  Sqrt : Sqrt
  Sqrt1 : Sqrt
  Transpose : Math  Operator=transpose
  m dot m : DotProduct  OutDataTypeStr=Inherit: Inherit via internal rule
  r dot m_master : DotProduct  OutDataTypeStr=Inherit: Inherit via internal rule
  r dot m_slave : DotProduct  OutDataTypeStr=Inherit: Inherit via internal rule
  Source_Torque : Outport
  Source_Force : Outport  Port=2
  wires:
  Power/1 -> Gain/1
  Transpose/1 -> Matrix Multiply/2
  Gain1/1 -> Add/1
  Matrix Multiply/1 -> Gain1/1
  Sqrt/1 -> Power/1
  Gain/1 -> Product/2
  Dot Product/1 -> Sqrt/1
  Product/1 -> Cross Product/2
  Matrix Multiply1/1 -> Product/1
  Normalize Vector/1 -> Transpose/1, Matrix Multiply/1
  IdentityMatrix/1 -> Add/2
  Constant/1 -> Power/2
  Add/1 -> Matrix Multiply1/1
  Slave_Pos/1 -> Add1/1
  Source_Pos/1 -> Add1/2
  Cross Product/1 -> Source_Torque/1
  Slave_Moment/1 -> Cross Product/1, Product2/2, m dot m/1, r dot m_slave/2
  Normalize Vector1/1 -> r dot m_slave/1, r dot m_master/1, Product4/2
  Add3/1 -> Product5/2
  Gain2/1 -> Product5/1
  Product4/1 -> Add3/3
  Dot Product1/1 -> Sqrt1/1
  Gain3/1 -> Add2/2
  r dot m_master/1 -> Product3/2, Product2/1
  Source_Moment/1 -> Matrix Multiply1/2, m dot m/2, Product1/2, r dot m_master/2
  m dot m/1 -> Add2/1
  Power1/1 -> Gain2/1
  Sqrt1/1 -> Power1/1
  r dot m_slave/1 -> Product1/1, Product3/1
  Product2/1 -> Add3/2
  Constant1/1 -> Power1/2
  Add2/1 -> Product4/1
  Add1/1 -> Normalize Vector1/1, Dot Product1/2, Dot Product1/1, Dot Product/2, Dot Product/1, Normalize Vector/1
  Product3/1 -> Gain3/1
  Product1/1 -> Add3/1
  Product5/1 -> Source_Force/1

== system Copy_of_tests/Multi-Arm system/Single_Arm 2/Plate_5/Torques and Forces ==
  m_slave : Inport
  Pos_Slave : Inport  Port=2
  M1 : Inport  Port=3
  Pos_Plate1 : Inport  Port=4
  M2 : Inport  Port=5
  Pos_Plate2 : Inport  Port=6
  M3 : Inport  Port=7
  Pos_Plate3 : Inport  Port=8
  M4 : Inport  Port=9
  Pos_Plate4 : Inport  Port=10
  M6 : Inport  Port=11
  Pos_Plate6 : Inport  Port=12
  Add{,1..4} (5 alike) : Sum  Inputs=+-
  Magnetic Forces : Subsystem
  Magnetic Torques : Subsystem
      settings: PortSchema="{\"entries\":[{\"content\":{\"sides\":[{\"content\":{\"connectorIds\":[\"In1\",\"In2\",\"In3\",\"In4\",\"In5\",\"In6\",\"In7\",\"In8\",\"In9\",\"In10\",\"In11\"]},\"type\":\"ConnectorPlacement.EquallySpacedRectSide\",\"uuid\":\"05771496-45a2-4580-b6ab-cadf9064ee26\"},{\"content\":{\"connectorIds\":[\"Out1\"],\"side\":\"RIGHT\"},\"type\":\"ConnectorPlacement.EquallySpacedRectSide\",\"uuid\":\"b79900f2-9f02-4790-af3a-0fbba66daa11\"},{\"content\":{\"connectorIds\":[\"LConn1\"],\"side\":\"TOP\"},\"type\":\"ConnectorPlacement.EquallySpacedRectSide\",\"uuid\":\"95266051-22b3-46d7-add2-de0ce2a92008\"}]},\"type\":\"ConnectorPlacement.EquallySpacedConnector\",\"uuid\":\"2bf1b23d-6512-437d-b945-3c726b6a255c\"}],\"packageUris\":[\"http://schema.mathworks.com/mf0/Connector/R2020b\"],\"version\":\"1.0\"}"
  brick reference : PMIOPort  Side=Left
  Forces : Outport
  Torques : Outport  Port=2
  wires:
  m_slave/1 -> Magnetic Forces/1(m_slave), Magnetic Torques/1(m_slave)
  Pos_Slave/1 -> Add4/1, Add3/1, Add2/1, Add1/1, Add/1
  Pos_Plate1/1 -> Add/2
  M1/1 -> Magnetic Torques/2(M1), Magnetic Forces/2(M1)
  Add/1 -> Magnetic Torques/7(r1), Magnetic Forces/7(r1)
  Pos_Plate6/1 -> Add4/2
  Pos_Plate4/1 -> Add3/2
  Pos_Plate3/1 -> Add2/2
  Pos_Plate2/1 -> Add1/2
  M2/1 -> Magnetic Forces/3(M2), Magnetic Torques/3(M2)
  Add1/1 -> Magnetic Torques/8(r2), Magnetic Forces/8(r2)
  M3/1 -> Magnetic Forces/4(M3), Magnetic Torques/4(M3)
  M4/1 -> Magnetic Forces/5(M4), Magnetic Torques/5(M4)
  M6/1 -> Magnetic Forces/6(M6), Magnetic Torques/6(M6)
  Add2/1 -> Magnetic Forces/9(r3), Magnetic Torques/9(r3)
  Add3/1 -> Magnetic Forces/10(r4), Magnetic Torques/10(r4)
  Add4/1 -> Magnetic Forces/11(r6), Magnetic Torques/11(r6)
  Magnetic Forces/1(Forces) -> Forces/1
  Magnetic Torques/1(Torque) -> Torques/1
  connections:
  brick reference/RConn1 -- Magnetic Torques/LConn1
